simulink model "model_oper_point_gaslift"  (R2023a)
settings: Solver=FixedStepAuto  StartTime=0.0  StopTime=100  FixedStep=0.1  RelTol=1e-3
values from neighbouring files (symbols this model uses):
  par = function_parameter_oper_point_gaslift    [main_oper_point_gaslift.m]    (also in workspace_oper_point_gaslift.mat = )
settings Model: Creator=aslik  LastModifiedBy=aslik

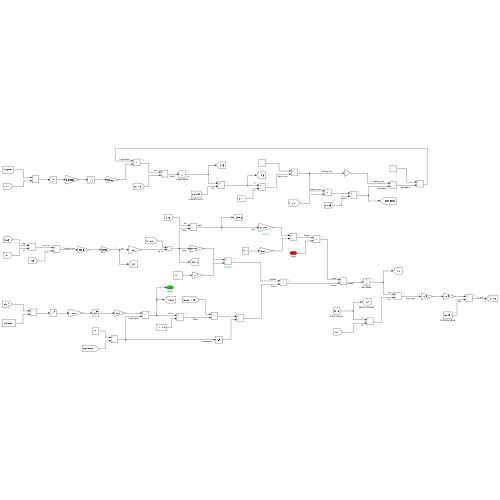
[thumbnail: Simulink's stored preview of the top-level diagram]
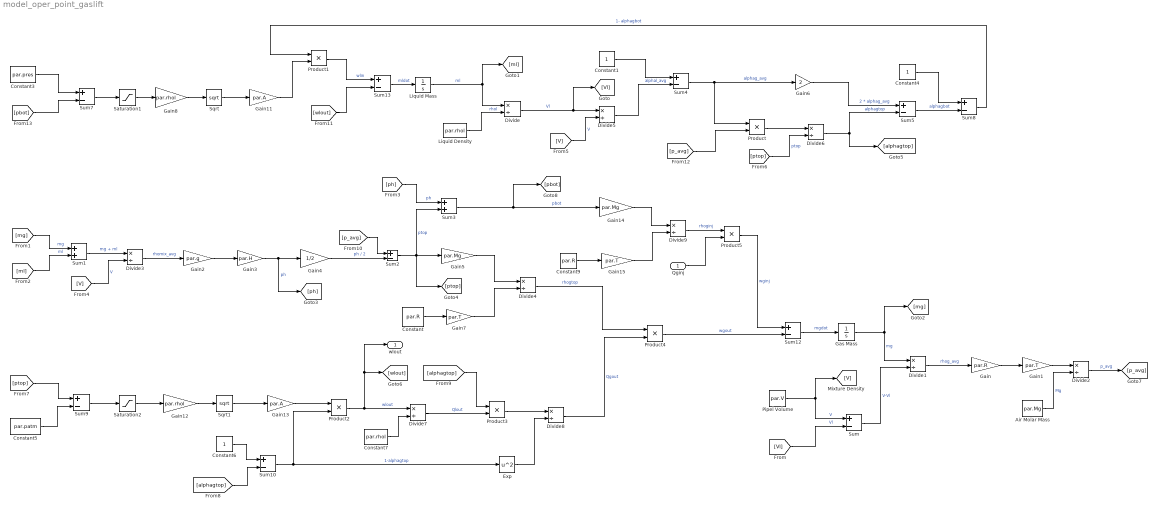
== system model_oper_point_gaslift ==
  Qginj : Inport
  Air Molar Mass : Constant  Value=par.Mg
  Constant : Constant  Value=par.R
  Constant1 : Constant
  Constant3 : Constant  Value=par.pres
  Constant4 : Constant
  Constant5 : Constant  Value=par.patm
  Constant6 : Constant
  Constant7 : Constant  Value=par.rhol
  Constant9 : Constant  Value=par.R
  Divide{,1..9} (10 alike) : Product  Inputs=*/
  Exp : Math  Operator=square
  Gain : Gain  Gain=par.R
  Gain1 : Gain  Gain=par.T
  Gain11 : Gain  Gain=par.A
  Gain12 : Gain  Gain=par.rhol
  Gain13 : Gain  Gain=par.A
  Gain14 : Gain  Gain=par.Mg
  Gain15 : Gain  Gain=par.T
  Gain2 : Gain  Gain=par.g
  Gain3 : Gain  Gain=par.H
  Gain4 : Gain  Gain=1/2
  Gain5 : Gain  Gain=par.Mg
  Gain6 : Gain  Gain=2
  Gain7 : Gain  Gain=par.T
  Gain8 : Gain  Gain=par.rhol
  "Gas Mass " : Integrator  InitialCondition=par.mg0  LowerSaturationLimit=0  ContinuousStateAttributes='mg'
  Liquid Density : Constant  Value=par.rhol
  Liquid Mass : Integrator  InitialCondition=par.ml0  LowerSaturationLimit=0  ContinuousStateAttributes='ml'
  Pipel Volume : Constant  Value=par.V
  Product{,1..5} (6 alike) : Product
  Saturation1 : Saturate  UpperLimit=inf  LowerLimit=0
  Saturation2 : Saturate  UpperLimit=inf  LowerLimit=0
  Sqrt : Sqrt
  Sqrt1 : Sqrt
  Sum{,2,4..5,7..10,12..13} (10 alike) : Sum  Inputs=+-
  Sum1 : Sum
  Sum3 : Sum
  wlout : Outport
  wires:
  Gain14/1 -> Divide9/1
  Gain15/1 -> Divide9/2
  Divide7/1 -> Product3/2  "Qlout"
  Constant/1 -> Gain7/1
  Constant7/1 -> Divide7/2
  Divide8/1 -> Product4/2  "Qgout"
  Sqrt1/1 -> Gain13/1
  Gain3/1 -> [ph], Gain4/1  "ph"
  Constant5/1 -> Sum9/2
  [ptop] -> Sum9/1
  [alphagtop] -> Sum10/2
  [V] -> Divide3/2  "V"
  Gain4/1 -> Sum2/2  "ph / 2"
  Product2/1 -> wlout/1, [wlout], Divide7/1  "wlout"
  Gain13/1 -> Product2/1
  Gain7/1 -> Divide4/2
  Sum12/1 -> "Gas Mass "/1  "mgdot"
  Gain5/1 -> Divide4/1
  [alphagtop] -> Product3/1
  [ml] -> Sum1/2  "ml"
  Qginj/1 -> Product5/2
  Constant9/1 -> Gain15/1
  Divide9/1 -> Product5/1  "rhoginj"
  Divide3/1 -> Gain2/1  "rhomix_avg"
  Divide4/1 -> Product4/1  "rhogtop"
  Product5/1 -> Sum12/1  "wginj"
  [ph] -> Sum3/1  "ph"
  Sum3/1 -> [pbot], Gain14/1  "pbot"
  Exp/1 -> Divide8/2
  Sum2/1 -> Gain5/1, Sum3/2, [ptop]  "ptop"
  Sum1/1 -> Divide3/1  "mg + ml"
  Product4/1 -> Sum12/2  "wgout"
  [mg] -> Sum1/1  "mg"
  Sum9/1 -> Saturation2/1
  Product3/1 -> Divide8/1
  Sum10/1 -> Product2/2, Exp/1  "1-alphagtop"
  Constant6/1 -> Sum10/1
  Gain2/1 -> Gain3/1
  Constant4/1 -> Sum8/1
  Sqrt/1 -> Gain11/1
  [V] -> Divide5/2  "V"
  Sum13/1 -> Liquid Mass/1  "mldot"
  Divide/1 -> Divide5/1, [Vl]  "Vl"
  Sum8/1 -> Product1/1  "1- alphagbot"
  [Vl] -> Sum/2  "Vl"
  Sum4/1 -> Product/1, Gain6/1  "alphag_avg"
  Gain1/1 -> Divide2/1
  Sum7/1 -> Saturation1/1
  Gain11/1 -> Product1/2
  Divide5/1 -> Sum4/2  "alphal_avg"
  Sum5/1 -> Sum8/2  "alphagbot"
  [ptop] -> Divide6/2  "ptop"
  Divide6/1 -> [alphagtop], Sum5/2  "alphagtop"
  Product/1 -> Divide6/1
  [wlout] -> Sum13/2
  Constant1/1 -> Sum4/1
  Divide1/1 -> Gain/1  "rhog_avg"
  Sum/1 -> Divide1/2  "V-Vl"
  Divide2/1 -> [p_avg]  "p_avg"
  Gain6/1 -> Sum5/1  "2 * alphag_avg"
  Liquid Mass/1 -> [ml], Divide/1  "ml"
  Product1/1 -> Sum13/1  "wlin"
  Liquid Density/1 -> Divide/2  "rhol"
  Pipel Volume/1 -> Sum/1, [V]  "V"
  Saturation1/1 -> Gain8/1
  Air Molar Mass/1 -> Divide2/2  "Mg"
  Gain/1 -> Gain1/1
  "Gas Mass "/1 -> [mg], Divide1/1  "mg"
  [p_avg] -> Sum2/1
  [p_avg] -> Product/2
  [pbot] -> Sum7/2
  Constant3/1 -> Sum7/1
  Gain8/1 -> Sqrt/1
  Gain12/1 -> Sqrt1/1
  Saturation2/1 -> Gain12/1
